simulink model "IntAdd"  (R2014a)
settings: Solver=ode45  StartTime=0.0  StopTime=10.0  RelTol=1e-3
settings Model: Creator=Shiyu  LastModifiedBy=Shiyu

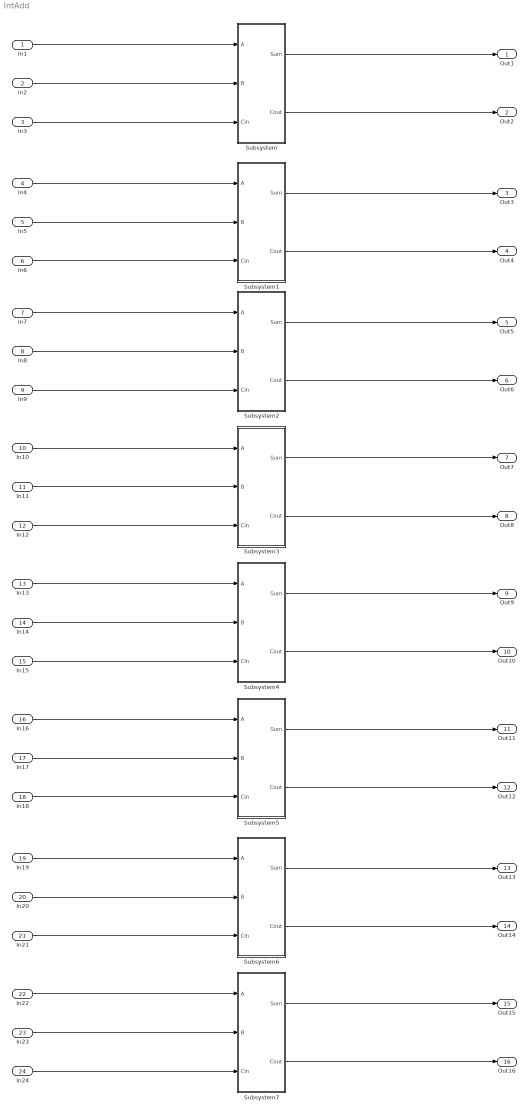
== system IntAdd ==
  In1 : Inport  OutDataTypeStr=boolean  SampleTime=1
  In2 : Inport  Port=2  OutDataTypeStr=boolean  SampleTime=1
  In3 : Inport  Port=3  OutDataTypeStr=boolean  SampleTime=1
  In4 : Inport  Port=4  OutDataTypeStr=boolean  SampleTime=1
  In5 : Inport  Port=5  OutDataTypeStr=boolean  SampleTime=1
  In6 : Inport  Port=6  OutDataTypeStr=boolean  SampleTime=1
  In7 : Inport  Port=7  OutDataTypeStr=boolean  SampleTime=1
  In8 : Inport  Port=8  OutDataTypeStr=boolean  SampleTime=1
  In9 : Inport  Port=9  OutDataTypeStr=boolean  SampleTime=1
  In10 : Inport  Port=10  OutDataTypeStr=boolean  SampleTime=1
  In11 : Inport  Port=11  OutDataTypeStr=boolean  SampleTime=1
  In12 : Inport  Port=12  OutDataTypeStr=boolean  SampleTime=1
  In13 : Inport  Port=13  OutDataTypeStr=boolean  SampleTime=1
  In14 : Inport  Port=14  OutDataTypeStr=boolean  SampleTime=1
  In15 : Inport  Port=15  OutDataTypeStr=boolean  SampleTime=1
  In16 : Inport  Port=16  OutDataTypeStr=boolean  SampleTime=1
  In17 : Inport  Port=17  OutDataTypeStr=boolean  SampleTime=1
  In18 : Inport  Port=18  OutDataTypeStr=boolean  SampleTime=1
  In19 : Inport  Port=19  OutDataTypeStr=boolean  SampleTime=1
  In20 : Inport  Port=20  OutDataTypeStr=boolean  SampleTime=1
  In21 : Inport  Port=21  OutDataTypeStr=boolean  SampleTime=1
  In22 : Inport  Port=22  OutDataTypeStr=boolean  SampleTime=1
  In23 : Inport  Port=23  OutDataTypeStr=boolean  SampleTime=1
  In24 : Inport  Port=24  OutDataTypeStr=boolean  SampleTime=1
  Subsystem : Subsystem
  Subsystem1 : Subsystem
  Subsystem2 : Subsystem
  Subsystem3 : Subsystem
  Subsystem4 : Subsystem
  Subsystem5 : Subsystem
  Subsystem6 : Subsystem
  Subsystem7 : Subsystem
  Out1 : Outport
  Out2 : Outport  Port=2
  Out3 : Outport  Port=3
  Out4 : Outport  Port=4
  Out5 : Outport  Port=5
  Out6 : Outport  Port=6
  Out7 : Outport  Port=7
  Out8 : Outport  Port=8
  Out9 : Outport  Port=9
  Out10 : Outport  Port=10
  Out11 : Outport  Port=11
  Out12 : Outport  Port=12
  Out13 : Outport  Port=13
  Out14 : Outport  Port=14
  Out15 : Outport  Port=15
  Out16 : Outport  Port=16
  wires:
  In1/1 -> Subsystem/1(A)
  In2/1 -> Subsystem/2(B)
  In3/1 -> Subsystem/3(Cin)
  Subsystem/1(Sum) -> Out1/1
  Subsystem/2(Cout) -> Out2/1
  In4/1 -> Subsystem1/1(A)
  In5/1 -> Subsystem1/2(B)
  In6/1 -> Subsystem1/3(Cin)
  Subsystem1/1(Sum) -> Out3/1
  Subsystem1/2(Cout) -> Out4/1
  In7/1 -> Subsystem2/1(A)
  In8/1 -> Subsystem2/2(B)
  In9/1 -> Subsystem2/3(Cin)
  Subsystem2/1(Sum) -> Out5/1
  Subsystem2/2(Cout) -> Out6/1
  In10/1 -> Subsystem3/1(A)
  In11/1 -> Subsystem3/2(B)
  In12/1 -> Subsystem3/3(Cin)
  Subsystem3/1(Sum) -> Out7/1
  Subsystem3/2(Cout) -> Out8/1
  In13/1 -> Subsystem4/1(A)
  In14/1 -> Subsystem4/2(B)
  In15/1 -> Subsystem4/3(Cin)
  Subsystem4/1(Sum) -> Out9/1
  Subsystem4/2(Cout) -> Out10/1
  In16/1 -> Subsystem5/1(A)
  In17/1 -> Subsystem5/2(B)
  In18/1 -> Subsystem5/3(Cin)
  Subsystem5/1(Sum) -> Out11/1
  Subsystem5/2(Cout) -> Out12/1
  In19/1 -> Subsystem6/1(A)
  In20/1 -> Subsystem6/2(B)
  In21/1 -> Subsystem6/3(Cin)
  Subsystem6/1(Sum) -> Out13/1
  Subsystem6/2(Cout) -> Out14/1
  In22/1 -> Subsystem7/1(A)
  In23/1 -> Subsystem7/2(B)
  In24/1 -> Subsystem7/3(Cin)
  Subsystem7/1(Sum) -> Out15/1
  Subsystem7/2(Cout) -> Out16/1

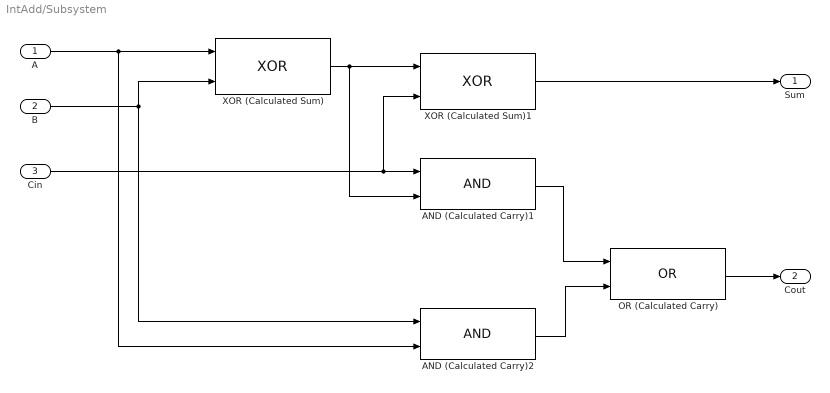
== system IntAdd/Subsystem ==
  A : Inport  OutDataTypeStr=boolean
  B : Inport  Port=2  OutDataTypeStr=boolean
  Cin : Inport  Port=3  OutDataTypeStr=boolean
  AND (Calculated Carry)1 : Logic  AllPortsSameDT=off  OutDataTypeStr=boolean
  AND (Calculated Carry)2 : Logic  AllPortsSameDT=off  OutDataTypeStr=boolean
  OR (Calculated Carry) : Logic  Operator=OR  AllPortsSameDT=off  OutDataTypeStr=boolean
  XOR (Calculated Sum) : Logic  Operator=XOR  AllPortsSameDT=off  OutDataTypeStr=boolean
  XOR (Calculated Sum)1 : Logic  Operator=XOR  AllPortsSameDT=off  OutDataTypeStr=boolean
  Sum : Outport
  Cout : Outport  Port=2
  wires:
  AND (Calculated Carry)1/1 -> OR (Calculated Carry)/1
  XOR (Calculated Sum)/1 -> AND (Calculated Carry)1/2, XOR (Calculated Sum)1/1
  OR (Calculated Carry)/1 -> Cout/1
  Cin/1 -> XOR (Calculated Sum)1/2, AND (Calculated Carry)1/1
  XOR (Calculated Sum)1/1 -> Sum/1
  A/1 -> AND (Calculated Carry)2/2, XOR (Calculated Sum)/1
  B/1 -> AND (Calculated Carry)2/1, XOR (Calculated Sum)/2
  AND (Calculated Carry)2/1 -> OR (Calculated Carry)/2

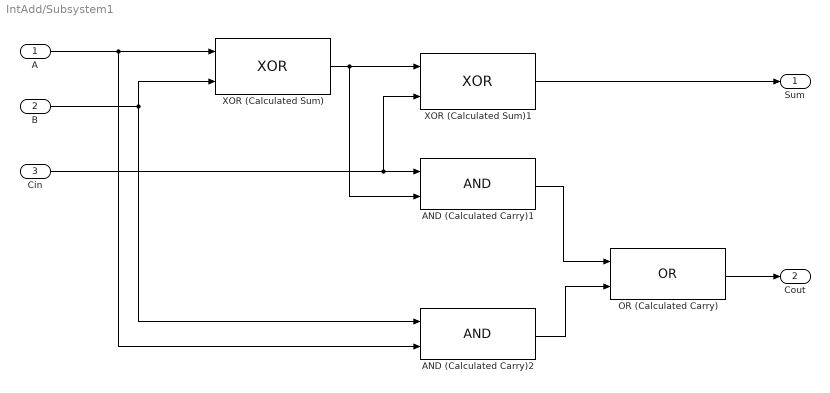
== system IntAdd/Subsystem1 ==
  A : Inport  OutDataTypeStr=boolean
  B : Inport  Port=2  OutDataTypeStr=boolean
  Cin : Inport  Port=3  OutDataTypeStr=boolean
  AND (Calculated Carry)1 : Logic  AllPortsSameDT=off  OutDataTypeStr=boolean
  AND (Calculated Carry)2 : Logic  AllPortsSameDT=off  OutDataTypeStr=boolean
  OR (Calculated Carry) : Logic  Operator=OR  AllPortsSameDT=off  OutDataTypeStr=boolean
  XOR (Calculated Sum) : Logic  Operator=XOR  AllPortsSameDT=off  OutDataTypeStr=boolean
  XOR (Calculated Sum)1 : Logic  Operator=XOR  AllPortsSameDT=off  OutDataTypeStr=boolean
  Sum : Outport
  Cout : Outport  Port=2
  wires:
  AND (Calculated Carry)1/1 -> OR (Calculated Carry)/1
  XOR (Calculated Sum)/1 -> AND (Calculated Carry)1/2, XOR (Calculated Sum)1/1
  OR (Calculated Carry)/1 -> Cout/1
  Cin/1 -> XOR (Calculated Sum)1/2, AND (Calculated Carry)1/1
  XOR (Calculated Sum)1/1 -> Sum/1
  A/1 -> AND (Calculated Carry)2/2, XOR (Calculated Sum)/1
  B/1 -> AND (Calculated Carry)2/1, XOR (Calculated Sum)/2
  AND (Calculated Carry)2/1 -> OR (Calculated Carry)/2

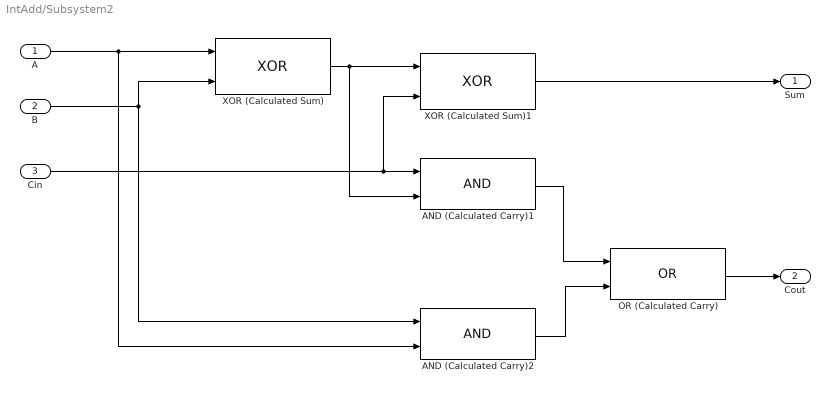
== system IntAdd/Subsystem2 ==
  A : Inport  OutDataTypeStr=boolean
  B : Inport  Port=2  OutDataTypeStr=boolean
  Cin : Inport  Port=3  OutDataTypeStr=boolean
  AND (Calculated Carry)1 : Logic  AllPortsSameDT=off  OutDataTypeStr=boolean
  AND (Calculated Carry)2 : Logic  AllPortsSameDT=off  OutDataTypeStr=boolean
  OR (Calculated Carry) : Logic  Operator=OR  AllPortsSameDT=off  OutDataTypeStr=boolean
  XOR (Calculated Sum) : Logic  Operator=XOR  AllPortsSameDT=off  OutDataTypeStr=boolean
  XOR (Calculated Sum)1 : Logic  Operator=XOR  AllPortsSameDT=off  OutDataTypeStr=boolean
  Sum : Outport
  Cout : Outport  Port=2
  wires:
  AND (Calculated Carry)1/1 -> OR (Calculated Carry)/1
  XOR (Calculated Sum)/1 -> AND (Calculated Carry)1/2, XOR (Calculated Sum)1/1
  OR (Calculated Carry)/1 -> Cout/1
  Cin/1 -> XOR (Calculated Sum)1/2, AND (Calculated Carry)1/1
  XOR (Calculated Sum)1/1 -> Sum/1
  A/1 -> AND (Calculated Carry)2/2, XOR (Calculated Sum)/1
  B/1 -> AND (Calculated Carry)2/1, XOR (Calculated Sum)/2
  AND (Calculated Carry)2/1 -> OR (Calculated Carry)/2

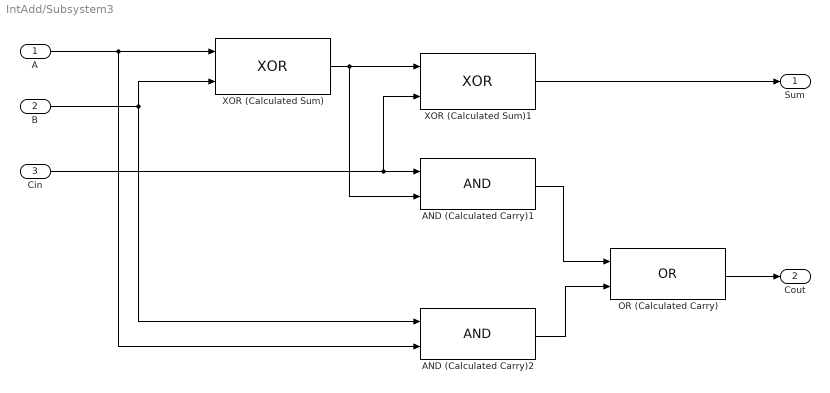
== system IntAdd/Subsystem3 ==
  A : Inport  OutDataTypeStr=boolean
  B : Inport  Port=2  OutDataTypeStr=boolean
  Cin : Inport  Port=3  OutDataTypeStr=boolean
  AND (Calculated Carry)1 : Logic  AllPortsSameDT=off  OutDataTypeStr=boolean
  AND (Calculated Carry)2 : Logic  AllPortsSameDT=off  OutDataTypeStr=boolean
  OR (Calculated Carry) : Logic  Operator=OR  AllPortsSameDT=off  OutDataTypeStr=boolean
  XOR (Calculated Sum) : Logic  Operator=XOR  AllPortsSameDT=off  OutDataTypeStr=boolean
  XOR (Calculated Sum)1 : Logic  Operator=XOR  AllPortsSameDT=off  OutDataTypeStr=boolean
  Sum : Outport
  Cout : Outport  Port=2
  wires:
  AND (Calculated Carry)1/1 -> OR (Calculated Carry)/1
  XOR (Calculated Sum)/1 -> AND (Calculated Carry)1/2, XOR (Calculated Sum)1/1
  OR (Calculated Carry)/1 -> Cout/1
  Cin/1 -> XOR (Calculated Sum)1/2, AND (Calculated Carry)1/1
  XOR (Calculated Sum)1/1 -> Sum/1
  A/1 -> AND (Calculated Carry)2/2, XOR (Calculated Sum)/1
  B/1 -> AND (Calculated Carry)2/1, XOR (Calculated Sum)/2
  AND (Calculated Carry)2/1 -> OR (Calculated Carry)/2

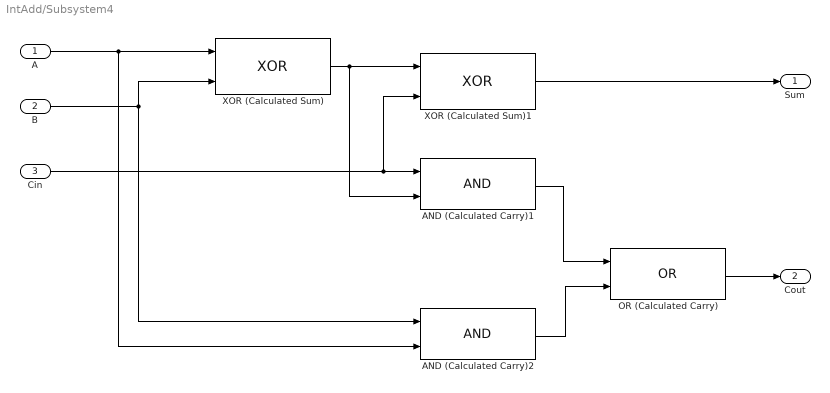
== system IntAdd/Subsystem4 ==
  A : Inport  OutDataTypeStr=boolean
  B : Inport  Port=2  OutDataTypeStr=boolean
  Cin : Inport  Port=3  OutDataTypeStr=boolean
  AND (Calculated Carry)1 : Logic  AllPortsSameDT=off  OutDataTypeStr=boolean
  AND (Calculated Carry)2 : Logic  AllPortsSameDT=off  OutDataTypeStr=boolean
  OR (Calculated Carry) : Logic  Operator=OR  AllPortsSameDT=off  OutDataTypeStr=boolean
  XOR (Calculated Sum) : Logic  Operator=XOR  AllPortsSameDT=off  OutDataTypeStr=boolean
  XOR (Calculated Sum)1 : Logic  Operator=XOR  AllPortsSameDT=off  OutDataTypeStr=boolean
  Sum : Outport
  Cout : Outport  Port=2
  wires:
  AND (Calculated Carry)1/1 -> OR (Calculated Carry)/1
  XOR (Calculated Sum)/1 -> AND (Calculated Carry)1/2, XOR (Calculated Sum)1/1
  OR (Calculated Carry)/1 -> Cout/1
  Cin/1 -> XOR (Calculated Sum)1/2, AND (Calculated Carry)1/1
  XOR (Calculated Sum)1/1 -> Sum/1
  A/1 -> AND (Calculated Carry)2/2, XOR (Calculated Sum)/1
  B/1 -> AND (Calculated Carry)2/1, XOR (Calculated Sum)/2
  AND (Calculated Carry)2/1 -> OR (Calculated Carry)/2

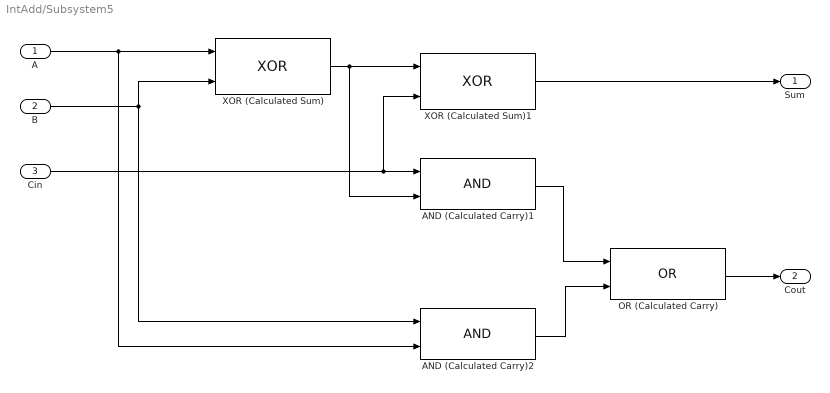
== system IntAdd/Subsystem5 ==
  A : Inport  OutDataTypeStr=boolean
  B : Inport  Port=2  OutDataTypeStr=boolean
  Cin : Inport  Port=3  OutDataTypeStr=boolean
  AND (Calculated Carry)1 : Logic  AllPortsSameDT=off  OutDataTypeStr=boolean
  AND (Calculated Carry)2 : Logic  AllPortsSameDT=off  OutDataTypeStr=boolean
  OR (Calculated Carry) : Logic  Operator=OR  AllPortsSameDT=off  OutDataTypeStr=boolean
  XOR (Calculated Sum) : Logic  Operator=XOR  AllPortsSameDT=off  OutDataTypeStr=boolean
  XOR (Calculated Sum)1 : Logic  Operator=XOR  AllPortsSameDT=off  OutDataTypeStr=boolean
  Sum : Outport
  Cout : Outport  Port=2
  wires:
  AND (Calculated Carry)1/1 -> OR (Calculated Carry)/1
  XOR (Calculated Sum)/1 -> AND (Calculated Carry)1/2, XOR (Calculated Sum)1/1
  OR (Calculated Carry)/1 -> Cout/1
  Cin/1 -> XOR (Calculated Sum)1/2, AND (Calculated Carry)1/1
  XOR (Calculated Sum)1/1 -> Sum/1
  A/1 -> AND (Calculated Carry)2/2, XOR (Calculated Sum)/1
  B/1 -> AND (Calculated Carry)2/1, XOR (Calculated Sum)/2
  AND (Calculated Carry)2/1 -> OR (Calculated Carry)/2

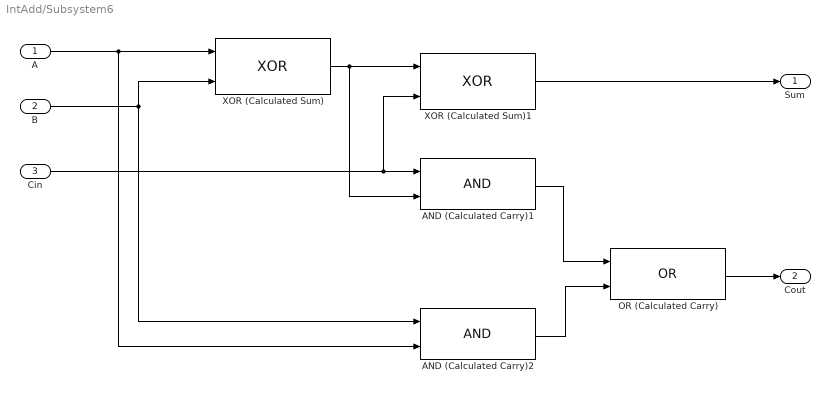
== system IntAdd/Subsystem6 ==
  A : Inport  OutDataTypeStr=boolean
  B : Inport  Port=2  OutDataTypeStr=boolean
  Cin : Inport  Port=3  OutDataTypeStr=boolean
  AND (Calculated Carry)1 : Logic  AllPortsSameDT=off  OutDataTypeStr=boolean
  AND (Calculated Carry)2 : Logic  AllPortsSameDT=off  OutDataTypeStr=boolean
  OR (Calculated Carry) : Logic  Operator=OR  AllPortsSameDT=off  OutDataTypeStr=boolean
  XOR (Calculated Sum) : Logic  Operator=XOR  AllPortsSameDT=off  OutDataTypeStr=boolean
  XOR (Calculated Sum)1 : Logic  Operator=XOR  AllPortsSameDT=off  OutDataTypeStr=boolean
  Sum : Outport
  Cout : Outport  Port=2
  wires:
  AND (Calculated Carry)1/1 -> OR (Calculated Carry)/1
  XOR (Calculated Sum)/1 -> AND (Calculated Carry)1/2, XOR (Calculated Sum)1/1
  OR (Calculated Carry)/1 -> Cout/1
  Cin/1 -> XOR (Calculated Sum)1/2, AND (Calculated Carry)1/1
  XOR (Calculated Sum)1/1 -> Sum/1
  A/1 -> AND (Calculated Carry)2/2, XOR (Calculated Sum)/1
  B/1 -> AND (Calculated Carry)2/1, XOR (Calculated Sum)/2
  AND (Calculated Carry)2/1 -> OR (Calculated Carry)/2

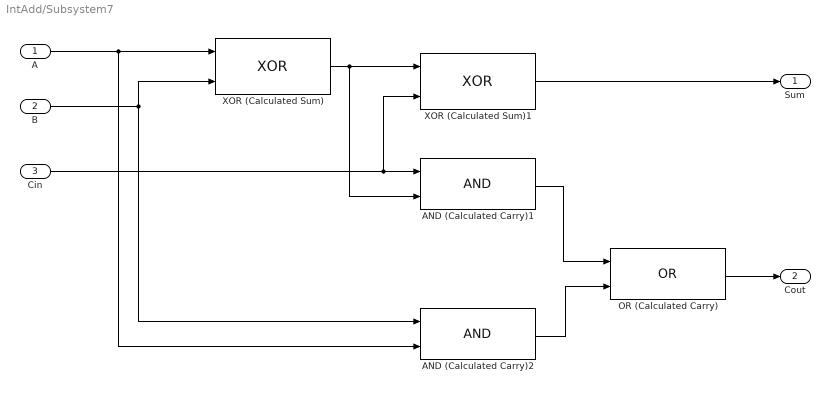
== system IntAdd/Subsystem7 ==
  A : Inport  OutDataTypeStr=boolean
  B : Inport  Port=2  OutDataTypeStr=boolean
  Cin : Inport  Port=3  OutDataTypeStr=boolean
  AND (Calculated Carry)1 : Logic  AllPortsSameDT=off  OutDataTypeStr=boolean
  AND (Calculated Carry)2 : Logic  AllPortsSameDT=off  OutDataTypeStr=boolean
  OR (Calculated Carry) : Logic  Operator=OR  AllPortsSameDT=off  OutDataTypeStr=boolean
  XOR (Calculated Sum) : Logic  Operator=XOR  AllPortsSameDT=off  OutDataTypeStr=boolean
  XOR (Calculated Sum)1 : Logic  Operator=XOR  AllPortsSameDT=off  OutDataTypeStr=boolean
  Sum : Outport
  Cout : Outport  Port=2
  wires:
  AND (Calculated Carry)1/1 -> OR (Calculated Carry)/1
  XOR (Calculated Sum)/1 -> AND (Calculated Carry)1/2, XOR (Calculated Sum)1/1
  OR (Calculated Carry)/1 -> Cout/1
  Cin/1 -> XOR (Calculated Sum)1/2, AND (Calculated Carry)1/1
  XOR (Calculated Sum)1/1 -> Sum/1
  A/1 -> AND (Calculated Carry)2/2, XOR (Calculated Sum)/1
  B/1 -> AND (Calculated Carry)2/1, XOR (Calculated Sum)/2
  AND (Calculated Carry)2/1 -> OR (Calculated Carry)/2
